simulink model "Prob_02"  (R2020a)
settings: Solver=VariableStepAuto  StartTime=0.0  StopTime=100  RelTol=1e-3
model workspace (MAT data in the model file):
  K1 = Simulink.Parameter
  K1.Value = 50
  K1.DataType = 'auto'
  K1.Dimensions = [1 1]
  K2 = Simulink.Parameter
  K2.Value = 20
  K2.DataType = 'auto'
  K2.Dimensions = [1 1]
  M1 = Simulink.Parameter
  M1.Value = 100
  M1.DataType = 'auto'
  M1.Dimensions = [1 1]
  M2 = Simulink.Parameter
  M2.Value = 10
  M2.DataType = 'auto'
  M2.Dimensions = [1 1]
  b = Simulink.Parameter
  b.Value = 50
  b.DataType = 'auto'
  b.Dimensions = [1 1]
settings Model: OrderedModelArguments=off  Creator=Shivam  LastModifiedBy=Shivam
settings DataIOCC: ExternalInput=x

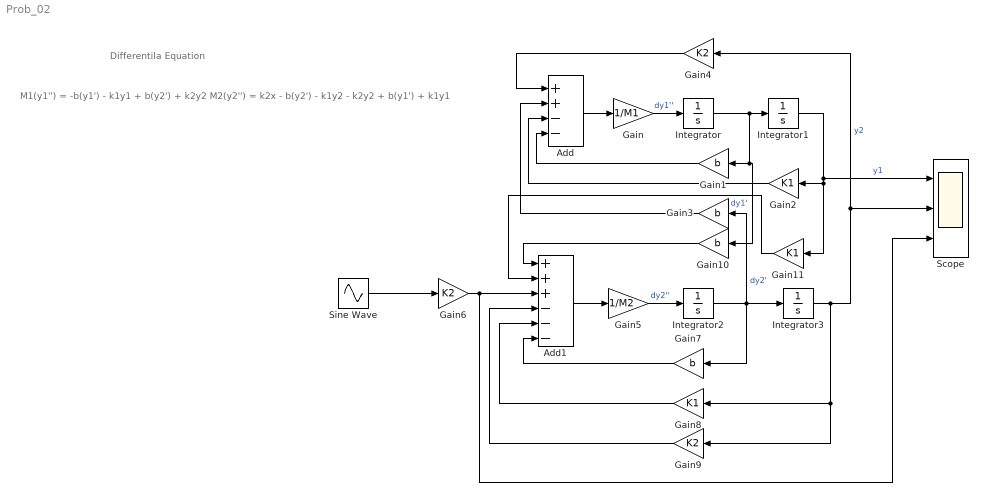
== system Prob_02 ==
  note: M1(y1'') = -b(y1') - k1y1 + b(y2') + k2y2
      |
      | M2(y2'') = k2x - b(y2') - k1y2 - k2y2 + b(y1') + k1y1
  note: Differentila Equation
  Add : Sum  Inputs=++--
  Add1 : Sum  Inputs=+++---
  Gain : Gain  Gain=1/M1
  Gain{1,3,7,10} (4 alike) : Gain  Gain=b
  Gain11 : Gain  Gain=K1
  Gain2 : Gain  Gain=K1
  Gain4 : Gain  Gain=K2
  Gain5 : Gain  Gain=1/M2
  Gain6 : Gain  Gain=K2
  Gain8 : Gain  Gain=K1
  Gain9 : Gain  Gain=K2
  Integrator{,1..3} (4 alike) : Integrator
  Scope : Scope  NumInputPorts=3
  Sine Wave : Sin  Amplitude=0.2  Frequency=0.2  SampleTime=0
  wires:
  Integrator/1 -> Gain1/1, Gain10/1, Integrator1/1  "dy1'"
  Integrator1/1 -> Gain2/1, Gain11/1, Scope/1  "y1"
  Integrator2/1 -> Gain7/1, Gain3/1, Integrator3/1  "dy2'"
  Integrator3/1 -> Gain9/1, Gain8/1, Scope/2, Gain4/1  "y2"
  Gain/1 -> Integrator/1  "dy1''"
  Add/1 -> Gain/1
  Gain1/1 -> Add/4
  Gain2/1 -> Add/3
  Gain3/1 -> Add/2
  Gain4/1 -> Add/1
  Gain5/1 -> Integrator2/1  "dy2''"
  Add1/1 -> Gain5/1
  Gain7/1 -> Add1/6
  Gain8/1 -> Add1/5
  Gain9/1 -> Add1/4
  Gain10/1 -> Add1/1
  Gain11/1 -> Add1/2
  Gain6/1 -> Scope/3, Add1/3
  Sine Wave/1 -> Gain6/1
